simulink model "indi_controller_tuning"  (R2024b)
settings: Solver=FixedStepAuto  StartTime=0.0  StopTime=inf  FixedStep=0.001  RelTol=1e-3
undefined symbols (not defined in the file): dirty_derivative, drawaircraft, drawaircraft2, dspblkCoreblockFVToolHelper, force_moment, gcbh, INDI, MAV, position_rhombus, reference_model, sample_time, SIM
libraries: slpidlib x12
(part 2 of 2)

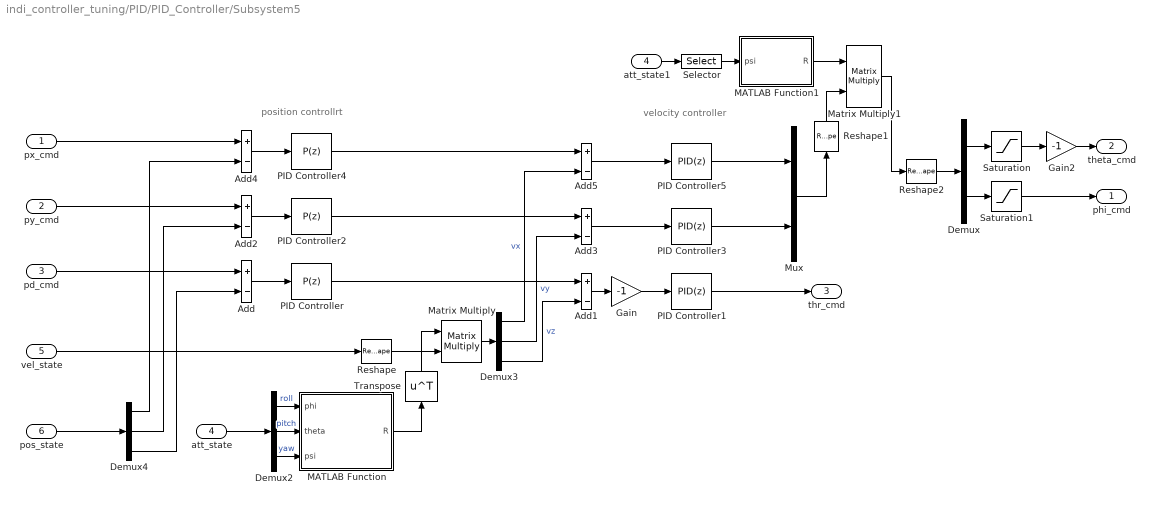
== system indi_controller_tuning/PID/PID_Controller/Subsystem5 ==
  note: velocity controller
  note: position controllrt
  px_cmd : Inport
  py_cmd : Inport  Port=2
  pd_cmd : Inport  Port=3
  att_state : Inport  Port=4
  vel_state : Inport  Port=5
  pos_state : Inport  Port=6
  Add{,1..5} (6 alike) : Sum  Inputs=+-
  Demux : Demux  Outputs=2
  Demux2 : Demux  Outputs=3
  Demux3 : Demux  Outputs=3
  Demux4 : Demux  Outputs=3
  Gain : Gain  Gain=-1
  Gain2 : Gain  Gain=-1
  MATLAB Function : MATLAB Function  TreatAsAtomicUnit=on
  MATLAB Function1 : MATLAB Function  TreatAsAtomicUnit=on
  Matrix Multiply : Product  Multiplication=Matrix(*)
  Matrix Multiply1 : Product  Multiplication=Matrix(*)
  Mux : Mux  Inputs=2
  PID Controller : slpidlib/PID Controller  Controller=P  Form=Parallel  TimeDomain=Discrete-time  UseExternalTs=off  SampleTime=sample_time  IntegratorMethod=Forward Euler  FilterMethod=Forward Euler  ControllerParametersSource=internal  P=1.55741678828513  I=1  UseKiTs=off  D=0  UseExternalDerivativeSource=off  N=100  UseFilter=on  TunerSelectOption=Transfer Function Based (PID Tuner App)  InitialConditionSource=internal  InitialConditionForIntegrator=0  InitialConditionForFilter=0  DifferentiatorICPrevScaledInput=0  ExternalReset=none  TrackingMode=off  Kt=1  LimitOutput=on  SatLimitsSource=internal  UpperSaturationLimit=2.5  LowerSaturationLimit=-2.5  LinearizeAsGain=on  AntiWindupMode=none  Kb=1  LimitIntegrator=off  UpperIntegratorSaturationLimit=inf  LowerIntegratorSaturationLimit=-inf  POutMin=[]  POutMax=[]  IOutMin=[]  IOutMax=[]  DOutMin=[]  DOutMax=[]  NOutMin=[]  NOutMax=[]  SumOutMin=[]  SumOutMax=[]  SaturationOutMin=[]  SaturationOutMax=[]  PParamMin=[]  PParamMax=[]  IParamMin=[]  IParamMax=[]  DParamMin=[]  DParamMax=[]  NParamMin=[]  NParamMax=[]  KbParamMin=[]  KbParamMax=[]  KtParamMin=[]  KtParamMax=[]  KbOutMin=[]  KbOutMax=[]  KtOutMin=[]  KtOutMax=[]  IntegratorOutMin=[]  IntegratorOutMax=[]  FilterOutMin=[]  FilterOutMax=[]  SumI1OutMin=[]  SumI1OutMax=[]  SumI2OutMin=[]  SumI2OutMax=[]  SumI3OutMin=[]  SumI3OutMax=[]  SumI4OutMin=[]  SumI4OutMax=[]  SumDOutMin=[]  SumDOutMax=[]  DifferentiatorOutMin=[]  DifferentiatorOutMax=[]  FilterDiffOutCoefMin=[]  FilterDiffOutCoefMax=[]  ReciprocalOutMin=[]  ReciprocalOutMax=[]  SumDenOutMin=[]  SumDenOutMax=[]  SumNumOutMin=[]  SumNumOutMax=[]  DivideOutMin=[]  DivideOutMax=[]  UdiffTsProdOutMin=[]  UdiffTsProdOutMax=[]  NTsProdOutMin=[]  NTsProdOutMax=[]  UintegralTsProdOutMin=[]  UintegralTsProdOutMax=[]  UngainTsProdOutMin=[]  UngainTsProdOutMax=[]  ClampingZeroOutDataTypeStr=Inherit: Inherit via back propagation  ClampingZeroOutMin=[]  ClampingZeroOutMax=[]  FilterDenConstantOutDataTypeStr=Inherit: Inherit via back propagation  FilterDenConstantOutMin=[]  FilterDenConstantOutMax=[]  PCopyOutDataTypeStr=Inherit: Inherit via back propagation  PCopyOutMin=[]  PCopyOutMax=[]  NCopyOutDataTypeStr=Inherit: Inherit via back propagation  NCopyOutMin=[]  NCopyOutMax=[]  IntegratorContinuousStateAttributes=''  IntegratorStateMustResolveToSignalObject=off  IntegratorRTWStateStorageClass=Auto  FilterContinuousStateAttributes=''  FilterStateMustResolveToSignalObject=off  FilterRTWStateStorageClass=Auto  ParallelPVariant=InternalParameters  IdealPVariant=Disabled  IVariant=Disabled  DVariant=Disabled  IntegratorVariant=Disabled  SatVariant=Enabled  AWVariant=Disabled  PCopyVariant=Disabled  TRVariant=Disabled  FdbkBlocksVariant=Forward  IdealPFdbkVariant=Disabled  SatFdbkVariant=Disabled  DerivativeFilterVariant=Disabled  NVariant=Disabled  NCopyVariant=Disabled_SignalSpec  FilterICVariant=Disabled  IntegratorICVariant=Disabled  ExternalResetVariant=Disabled  TRSumVariant=Passthrough  SumFdbkVariant=Disabled  SumVariant=Passthrough_P  TsampFilterVariant=InternalTs  TsampNgainVariant=Passthrough  TsampIntegralVariant=Disabled_SignalSpec  ExternalSaturationOutDataTypeStr=Inherit: Same as second input  DerivativeSourceVariant=Disabled  PreIntVariant=InternalPreInt
  PID Controller1 : slpidlib/PID Controller  Controller=PID  Form=Parallel  TimeDomain=Discrete-time  UseExternalTs=off  SampleTime=sample_time  IntegratorMethod=Forward Euler  FilterMethod=Forward Euler  ControllerParametersSource=internal  P=8.52067722160773  I=8.12576415570105  UseKiTs=off  D=0.164011038210978  UseExternalDerivativeSource=off  N=48.9353550982802  UseFilter=on  TunerSelectOption=Transfer Function Based (PID Tuner App)  InitialConditionSource=internal  InitialConditionForIntegrator=0  InitialConditionForFilter=0  DifferentiatorICPrevScaledInput=0  ExternalReset=none  TrackingMode=off  Kt=1  LimitOutput=on  SatLimitsSource=internal  UpperSaturationLimit=0.3*11  LowerSaturationLimit=-0.3*11  LinearizeAsGain=on  AntiWindupMode=clamping  Kb=1  LimitIntegrator=off  UpperIntegratorSaturationLimit=inf  LowerIntegratorSaturationLimit=-inf  POutMin=[]  POutMax=[]  IOutMin=[]  IOutMax=[]  DOutMin=[]  DOutMax=[]  NOutMin=[]  NOutMax=[]  SumOutMin=[]  SumOutMax=[]  SaturationOutMin=[]  SaturationOutMax=[]  PParamMin=[]  PParamMax=[]  IParamMin=[]  IParamMax=[]  DParamMin=[]  DParamMax=[]  NParamMin=[]  NParamMax=[]  KbParamMin=[]  KbParamMax=[]  KtParamMin=[]  KtParamMax=[]  KbOutMin=[]  KbOutMax=[]  KtOutMin=[]  KtOutMax=[]  IntegratorOutMin=[]  IntegratorOutMax=[]  FilterOutMin=[]  FilterOutMax=[]  SumI1OutMin=[]  SumI1OutMax=[]  SumI2OutMin=[]  SumI2OutMax=[]  SumI3OutMin=[]  SumI3OutMax=[]  SumI4OutMin=[]  SumI4OutMax=[]  SumDOutMin=[]  SumDOutMax=[]  DifferentiatorOutMin=[]  DifferentiatorOutMax=[]  FilterDiffOutCoefMin=[]  FilterDiffOutCoefMax=[]  ReciprocalOutMin=[]  ReciprocalOutMax=[]  SumDenOutMin=[]  SumDenOutMax=[]  SumNumOutMin=[]  SumNumOutMax=[]  DivideOutMin=[]  DivideOutMax=[]  UdiffTsProdOutMin=[]  UdiffTsProdOutMax=[]  NTsProdOutMin=[]  NTsProdOutMax=[]  UintegralTsProdOutMin=[]  UintegralTsProdOutMax=[]  UngainTsProdOutMin=[]  UngainTsProdOutMax=[]  ClampingZeroOutDataTypeStr=Inherit: Inherit via back propagation  ClampingZeroOutMin=[]  ClampingZeroOutMax=[]  FilterDenConstantOutDataTypeStr=Inherit: Inherit via back propagation  FilterDenConstantOutMin=[]  FilterDenConstantOutMax=[]  PCopyOutDataTypeStr=Inherit: Inherit via back propagation  PCopyOutMin=[]  PCopyOutMax=[]  NCopyOutDataTypeStr=Inherit: Inherit via back propagation  NCopyOutMin=[]  NCopyOutMax=[]  IntegratorContinuousStateAttributes=''  IntegratorStateMustResolveToSignalObject=off  IntegratorRTWStateStorageClass=Auto  FilterContinuousStateAttributes=''  FilterStateMustResolveToSignalObject=off  FilterRTWStateStorageClass=Auto  ParallelPVariant=InternalParameters  IdealPVariant=Disabled  IVariant=InternalParameters  DVariant=InternalParameters  IntegratorVariant=Discrete  SatVariant=Enabled  AWVariant=DiscClampingParallel  PCopyVariant=Disabled  TRVariant=Disabled  FdbkBlocksVariant=Forward  IdealPFdbkVariant=Disabled  SatFdbkVariant=Disabled  DerivativeFilterVariant=ForwardEulerFilter  NVariant=InternalParameters  NCopyVariant=Disabled  FilterICVariant=InternalICsFilter  IntegratorICVariant=InternalICs  ExternalResetVariant=Disabled  TRSumVariant=Passthrough  SumFdbkVariant=Disabled  SumVariant=Sum_PID  TsampFilterVariant=InternalTs  TsampNgainVariant=Passthrough  TsampIntegralVariant=Disabled_SignalSpec  ExternalSaturationOutDataTypeStr=Inherit: Same as second input  DerivativeSourceVariant=ErrorSignal  PreIntVariant=InternalPreInt
  PID Controller2 : slpidlib/PID Controller  Controller=P  Form=Parallel  TimeDomain=Discrete-time  UseExternalTs=off  SampleTime=sample_time  IntegratorMethod=Forward Euler  FilterMethod=Forward Euler  ControllerParametersSource=internal  P=0.183831516601899  I=1  UseKiTs=off  D=0  UseExternalDerivativeSource=off  N=100  UseFilter=on  TunerSelectOption=Transfer Function Based (PID Tuner App)  InitialConditionSource=internal  InitialConditionForIntegrator=0  InitialConditionForFilter=0  DifferentiatorICPrevScaledInput=0  ExternalReset=none  TrackingMode=off  Kt=1  LimitOutput=on  SatLimitsSource=internal  UpperSaturationLimit=5  LowerSaturationLimit=-5  LinearizeAsGain=on  AntiWindupMode=none  Kb=1  LimitIntegrator=off  UpperIntegratorSaturationLimit=inf  LowerIntegratorSaturationLimit=-inf  POutMin=[]  POutMax=[]  IOutMin=[]  IOutMax=[]  DOutMin=[]  DOutMax=[]  NOutMin=[]  NOutMax=[]  SumOutMin=[]  SumOutMax=[]  SaturationOutMin=[]  SaturationOutMax=[]  PParamMin=[]  PParamMax=[]  IParamMin=[]  IParamMax=[]  DParamMin=[]  DParamMax=[]  NParamMin=[]  NParamMax=[]  KbParamMin=[]  KbParamMax=[]  KtParamMin=[]  KtParamMax=[]  KbOutMin=[]  KbOutMax=[]  KtOutMin=[]  KtOutMax=[]  IntegratorOutMin=[]  IntegratorOutMax=[]  FilterOutMin=[]  FilterOutMax=[]  SumI1OutMin=[]  SumI1OutMax=[]  SumI2OutMin=[]  SumI2OutMax=[]  SumI3OutMin=[]  SumI3OutMax=[]  SumI4OutMin=[]  SumI4OutMax=[]  SumDOutMin=[]  SumDOutMax=[]  DifferentiatorOutMin=[]  DifferentiatorOutMax=[]  FilterDiffOutCoefMin=[]  FilterDiffOutCoefMax=[]  ReciprocalOutMin=[]  ReciprocalOutMax=[]  SumDenOutMin=[]  SumDenOutMax=[]  SumNumOutMin=[]  SumNumOutMax=[]  DivideOutMin=[]  DivideOutMax=[]  UdiffTsProdOutMin=[]  UdiffTsProdOutMax=[]  NTsProdOutMin=[]  NTsProdOutMax=[]  UintegralTsProdOutMin=[]  UintegralTsProdOutMax=[]  UngainTsProdOutMin=[]  UngainTsProdOutMax=[]  ClampingZeroOutDataTypeStr=Inherit: Inherit via back propagation  ClampingZeroOutMin=[]  ClampingZeroOutMax=[]  FilterDenConstantOutDataTypeStr=Inherit: Inherit via back propagation  FilterDenConstantOutMin=[]  FilterDenConstantOutMax=[]  PCopyOutDataTypeStr=Inherit: Inherit via back propagation  PCopyOutMin=[]  PCopyOutMax=[]  NCopyOutDataTypeStr=Inherit: Inherit via back propagation  NCopyOutMin=[]  NCopyOutMax=[]  IntegratorContinuousStateAttributes=''  IntegratorStateMustResolveToSignalObject=off  IntegratorRTWStateStorageClass=Auto  FilterContinuousStateAttributes=''  FilterStateMustResolveToSignalObject=off  FilterRTWStateStorageClass=Auto  ParallelPVariant=InternalParameters  IdealPVariant=Disabled  IVariant=Disabled  DVariant=Disabled  IntegratorVariant=Disabled  SatVariant=Enabled  AWVariant=Disabled  PCopyVariant=Disabled  TRVariant=Disabled  FdbkBlocksVariant=Forward  IdealPFdbkVariant=Disabled  SatFdbkVariant=Disabled  DerivativeFilterVariant=Disabled  NVariant=Disabled  NCopyVariant=Disabled_SignalSpec  FilterICVariant=Disabled  IntegratorICVariant=Disabled  ExternalResetVariant=Disabled  TRSumVariant=Passthrough  SumFdbkVariant=Disabled  SumVariant=Passthrough_P  TsampFilterVariant=InternalTs  TsampNgainVariant=Passthrough  TsampIntegralVariant=Disabled_SignalSpec  ExternalSaturationOutDataTypeStr=Inherit: Same as second input  DerivativeSourceVariant=Disabled  PreIntVariant=InternalPreInt
  PID Controller3 : slpidlib/PID Controller  Controller=PID  Form=Parallel  TimeDomain=Discrete-time  UseExternalTs=off  SampleTime=sample_time  IntegratorMethod=Forward Euler  FilterMethod=Forward Euler  ControllerParametersSource=internal  P=0.0381310436212984  I=0.0014813668367107  UseKiTs=off  D=-0.018399108574611  UseExternalDerivativeSource=off  N=1.45342970874378  UseFilter=on  TunerSelectOption=Transfer Function Based (PID Tuner App)  InitialConditionSource=internal  InitialConditionForIntegrator=0  InitialConditionForFilter=0  DifferentiatorICPrevScaledInput=0  ExternalReset=none  TrackingMode=off  Kt=1  LimitOutput=on  SatLimitsSource=internal  UpperSaturationLimit=deg2rad(8)  LowerSaturationLimit=-deg2rad(8)  LinearizeAsGain=on  AntiWindupMode=clamping  Kb=1  LimitIntegrator=off  UpperIntegratorSaturationLimit=inf  LowerIntegratorSaturationLimit=-inf  RndMeth=Ceiling  POutMin=[]  POutMax=[]  IOutMin=[]  IOutMax=[]  DOutMin=[]  DOutMax=[]  NOutMin=[]  NOutMax=[]  SumOutMin=[]  SumOutMax=[]  SaturationOutMin=[]  SaturationOutMax=[]  PParamMin=[]  PParamMax=[]  IParamMin=[]  IParamMax=[]  DParamMin=[]  DParamMax=[]  NParamMin=[]  NParamMax=[]  KbParamMin=[]  KbParamMax=[]  KtParamMin=[]  KtParamMax=[]  KbOutMin=[]  KbOutMax=[]  KtOutMin=[]  KtOutMax=[]  IntegratorOutMin=[]  IntegratorOutMax=[]  FilterOutMin=[]  FilterOutMax=[]  SumI1OutMin=[]  SumI1OutMax=[]  SumI2OutMin=[]  SumI2OutMax=[]  SumI3OutMin=[]  SumI3OutMax=[]  SumI4OutMin=[]  SumI4OutMax=[]  SumDOutMin=[]  SumDOutMax=[]  DifferentiatorOutMin=[]  DifferentiatorOutMax=[]  FilterDiffOutCoefMin=[]  FilterDiffOutCoefMax=[]  ReciprocalOutMin=[]  ReciprocalOutMax=[]  SumDenOutMin=[]  SumDenOutMax=[]  SumNumOutMin=[]  SumNumOutMax=[]  DivideOutMin=[]  DivideOutMax=[]  UdiffTsProdOutMin=[]  UdiffTsProdOutMax=[]  NTsProdOutMin=[]  NTsProdOutMax=[]  UintegralTsProdOutMin=[]  UintegralTsProdOutMax=[]  UngainTsProdOutMin=[]  UngainTsProdOutMax=[]  ClampingZeroOutDataTypeStr=Inherit: Inherit via back propagation  ClampingZeroOutMin=[]  ClampingZeroOutMax=[]  FilterDenConstantOutDataTypeStr=Inherit: Inherit via back propagation  FilterDenConstantOutMin=[]  FilterDenConstantOutMax=[]  PCopyOutDataTypeStr=Inherit: Inherit via back propagation  PCopyOutMin=[]  PCopyOutMax=[]  NCopyOutDataTypeStr=Inherit: Inherit via back propagation  NCopyOutMin=[]  NCopyOutMax=[]  IntegratorContinuousStateAttributes=''  IntegratorStateMustResolveToSignalObject=off  IntegratorRTWStateStorageClass=Auto  FilterContinuousStateAttributes=''  FilterStateMustResolveToSignalObject=off  FilterRTWStateStorageClass=Auto  ParallelPVariant=InternalParameters  IdealPVariant=Disabled  IVariant=InternalParameters  DVariant=InternalParameters  IntegratorVariant=Discrete  SatVariant=Enabled  AWVariant=DiscClampingParallel  PCopyVariant=Disabled  TRVariant=Disabled  FdbkBlocksVariant=Forward  IdealPFdbkVariant=Disabled  SatFdbkVariant=Disabled  DerivativeFilterVariant=ForwardEulerFilter  NVariant=InternalParameters  NCopyVariant=Disabled  FilterICVariant=InternalICsFilter  IntegratorICVariant=InternalICs  ExternalResetVariant=Disabled  TRSumVariant=Passthrough  SumFdbkVariant=Disabled  SumVariant=Sum_PID  TsampFilterVariant=InternalTs  TsampNgainVariant=Passthrough  TsampIntegralVariant=Disabled_SignalSpec  ExternalSaturationOutDataTypeStr=Inherit: Same as second input  DerivativeSourceVariant=ErrorSignal  PreIntVariant=InternalPreInt
  PID Controller4 : slpidlib/PID Controller  Controller=P  Form=Parallel  TimeDomain=Discrete-time  UseExternalTs=off  SampleTime=sample_time  IntegratorMethod=Forward Euler  FilterMethod=Forward Euler  ControllerParametersSource=internal  P=0.183831516601899  I=1  UseKiTs=off  D=0  UseExternalDerivativeSource=off  N=100  UseFilter=on  TunerSelectOption=Transfer Function Based (PID Tuner App)  InitialConditionSource=internal  InitialConditionForIntegrator=0  InitialConditionForFilter=0  DifferentiatorICPrevScaledInput=0  ExternalReset=none  TrackingMode=off  Kt=1  LimitOutput=on  SatLimitsSource=internal  UpperSaturationLimit=5  LowerSaturationLimit=-5  LinearizeAsGain=on  AntiWindupMode=none  Kb=1  LimitIntegrator=off  UpperIntegratorSaturationLimit=inf  LowerIntegratorSaturationLimit=-inf  POutMin=[]  POutMax=[]  IOutMin=[]  IOutMax=[]  DOutMin=[]  DOutMax=[]  NOutMin=[]  NOutMax=[]  SumOutMin=[]  SumOutMax=[]  SaturationOutMin=[]  SaturationOutMax=[]  PParamMin=[]  PParamMax=[]  IParamMin=[]  IParamMax=[]  DParamMin=[]  DParamMax=[]  NParamMin=[]  NParamMax=[]  KbParamMin=[]  KbParamMax=[]  KtParamMin=[]  KtParamMax=[]  KbOutMin=[]  KbOutMax=[]  KtOutMin=[]  KtOutMax=[]  IntegratorOutMin=[]  IntegratorOutMax=[]  FilterOutMin=[]  FilterOutMax=[]  SumI1OutMin=[]  SumI1OutMax=[]  SumI2OutMin=[]  SumI2OutMax=[]  SumI3OutMin=[]  SumI3OutMax=[]  SumI4OutMin=[]  SumI4OutMax=[]  SumDOutMin=[]  SumDOutMax=[]  DifferentiatorOutMin=[]  DifferentiatorOutMax=[]  FilterDiffOutCoefMin=[]  FilterDiffOutCoefMax=[]  ReciprocalOutMin=[]  ReciprocalOutMax=[]  SumDenOutMin=[]  SumDenOutMax=[]  SumNumOutMin=[]  SumNumOutMax=[]  DivideOutMin=[]  DivideOutMax=[]  UdiffTsProdOutMin=[]  UdiffTsProdOutMax=[]  NTsProdOutMin=[]  NTsProdOutMax=[]  UintegralTsProdOutMin=[]  UintegralTsProdOutMax=[]  UngainTsProdOutMin=[]  UngainTsProdOutMax=[]  ClampingZeroOutDataTypeStr=Inherit: Inherit via back propagation  ClampingZeroOutMin=[]  ClampingZeroOutMax=[]  FilterDenConstantOutDataTypeStr=Inherit: Inherit via back propagation  FilterDenConstantOutMin=[]  FilterDenConstantOutMax=[]  PCopyOutDataTypeStr=Inherit: Inherit via back propagation  PCopyOutMin=[]  PCopyOutMax=[]  NCopyOutDataTypeStr=Inherit: Inherit via back propagation  NCopyOutMin=[]  NCopyOutMax=[]  IntegratorContinuousStateAttributes=''  IntegratorStateMustResolveToSignalObject=off  IntegratorRTWStateStorageClass=Auto  FilterContinuousStateAttributes=''  FilterStateMustResolveToSignalObject=off  FilterRTWStateStorageClass=Auto  ParallelPVariant=InternalParameters  IdealPVariant=Disabled  IVariant=Disabled  DVariant=Disabled  IntegratorVariant=Disabled  SatVariant=Enabled  AWVariant=Disabled  PCopyVariant=Disabled  TRVariant=Disabled  FdbkBlocksVariant=Forward  IdealPFdbkVariant=Disabled  SatFdbkVariant=Disabled  DerivativeFilterVariant=Disabled  NVariant=Disabled  NCopyVariant=Disabled_SignalSpec  FilterICVariant=Disabled  IntegratorICVariant=Disabled  ExternalResetVariant=Disabled  TRSumVariant=Passthrough  SumFdbkVariant=Disabled  SumVariant=Passthrough_P  TsampFilterVariant=InternalTs  TsampNgainVariant=Passthrough  TsampIntegralVariant=Disabled_SignalSpec  ExternalSaturationOutDataTypeStr=Inherit: Same as second input  DerivativeSourceVariant=Disabled  PreIntVariant=InternalPreInt
  PID Controller5 : slpidlib/PID Controller  Controller=PID  Form=Parallel  TimeDomain=Discrete-time  UseExternalTs=off  SampleTime=sample_time  IntegratorMethod=Forward Euler  FilterMethod=Forward Euler  ControllerParametersSource=internal  P=0.0381310436212984  I=0.0014813668367107  UseKiTs=off  D=-0.018399108574611  UseExternalDerivativeSource=off  N=1.45342970874378  UseFilter=on  TunerSelectOption=Transfer Function Based (PID Tuner App)  InitialConditionSource=internal  InitialConditionForIntegrator=0  InitialConditionForFilter=0  DifferentiatorICPrevScaledInput=0  ExternalReset=none  TrackingMode=off  Kt=1  LimitOutput=on  SatLimitsSource=internal  UpperSaturationLimit=deg2rad(8)  LowerSaturationLimit=-deg2rad(8)  LinearizeAsGain=on  AntiWindupMode=clamping  Kb=1  LimitIntegrator=off  UpperIntegratorSaturationLimit=inf  LowerIntegratorSaturationLimit=-inf  RndMeth=Ceiling  POutMin=[]  POutMax=[]  IOutMin=[]  IOutMax=[]  DOutMin=[]  DOutMax=[]  NOutMin=[]  NOutMax=[]  SumOutMin=[]  SumOutMax=[]  SaturationOutMin=[]  SaturationOutMax=[]  PParamMin=[]  PParamMax=[]  IParamMin=[]  IParamMax=[]  DParamMin=[]  DParamMax=[]  NParamMin=[]  NParamMax=[]  KbParamMin=[]  KbParamMax=[]  KtParamMin=[]  KtParamMax=[]  KbOutMin=[]  KbOutMax=[]  KtOutMin=[]  KtOutMax=[]  IntegratorOutMin=[]  IntegratorOutMax=[]  FilterOutMin=[]  FilterOutMax=[]  SumI1OutMin=[]  SumI1OutMax=[]  SumI2OutMin=[]  SumI2OutMax=[]  SumI3OutMin=[]  SumI3OutMax=[]  SumI4OutMin=[]  SumI4OutMax=[]  SumDOutMin=[]  SumDOutMax=[]  DifferentiatorOutMin=[]  DifferentiatorOutMax=[]  FilterDiffOutCoefMin=[]  FilterDiffOutCoefMax=[]  ReciprocalOutMin=[]  ReciprocalOutMax=[]  SumDenOutMin=[]  SumDenOutMax=[]  SumNumOutMin=[]  SumNumOutMax=[]  DivideOutMin=[]  DivideOutMax=[]  UdiffTsProdOutMin=[]  UdiffTsProdOutMax=[]  NTsProdOutMin=[]  NTsProdOutMax=[]  UintegralTsProdOutMin=[]  UintegralTsProdOutMax=[]  UngainTsProdOutMin=[]  UngainTsProdOutMax=[]  ClampingZeroOutDataTypeStr=Inherit: Inherit via back propagation  ClampingZeroOutMin=[]  ClampingZeroOutMax=[]  FilterDenConstantOutDataTypeStr=Inherit: Inherit via back propagation  FilterDenConstantOutMin=[]  FilterDenConstantOutMax=[]  PCopyOutDataTypeStr=Inherit: Inherit via back propagation  PCopyOutMin=[]  PCopyOutMax=[]  NCopyOutDataTypeStr=Inherit: Inherit via back propagation  NCopyOutMin=[]  NCopyOutMax=[]  IntegratorContinuousStateAttributes=''  IntegratorStateMustResolveToSignalObject=off  IntegratorRTWStateStorageClass=Auto  FilterContinuousStateAttributes=''  FilterStateMustResolveToSignalObject=off  FilterRTWStateStorageClass=Auto  ParallelPVariant=InternalParameters  IdealPVariant=Disabled  IVariant=InternalParameters  DVariant=InternalParameters  IntegratorVariant=Discrete  SatVariant=Enabled  AWVariant=DiscClampingParallel  PCopyVariant=Disabled  TRVariant=Disabled  FdbkBlocksVariant=Forward  IdealPFdbkVariant=Disabled  SatFdbkVariant=Disabled  DerivativeFilterVariant=ForwardEulerFilter  NVariant=InternalParameters  NCopyVariant=Disabled  FilterICVariant=InternalICsFilter  IntegratorICVariant=InternalICs  ExternalResetVariant=Disabled  TRSumVariant=Passthrough  SumFdbkVariant=Disabled  SumVariant=Sum_PID  TsampFilterVariant=InternalTs  TsampNgainVariant=Passthrough  TsampIntegralVariant=Disabled_SignalSpec  ExternalSaturationOutDataTypeStr=Inherit: Same as second input  DerivativeSourceVariant=ErrorSignal  PreIntVariant=InternalPreInt
  Reshape : Reshape  OutputDimensionality=Column vector (2-D)
  Reshape1 : Reshape  OutputDimensionality=Column vector (2-D)
  Reshape2 : Reshape  OutputDimensionality=Row vector (2-D)
  Saturation : Saturate  UpperLimit=deg2rad(6)  LowerLimit=-deg2rad(6)
  Saturation1 : Saturate  UpperLimit=deg2rad(6)  LowerLimit=-deg2rad(6)
  Selector : Selector  InputPortWidth=3  IndexOptions=Index vector (dialog)  Indices=[3]  OutputSizes=1
  Transpose : Math  Operator=transpose
  att_state1 : InportShadow  Port=4
  phi_cmd : Outport
  theta_cmd : Outport  Port=2
  thr_cmd : Outport  Port=3
  wires:
  Reshape/1 -> Matrix Multiply/2
  Demux3/3 -> Add1/2  "vz"
  Matrix Multiply/1 -> Demux3/1
  MATLAB Function/1(R) -> Transpose/1
  Add1/1 -> Gain/1
  Transpose/1 -> Matrix Multiply/1
  Demux2/1 -> MATLAB Function/1(phi)  "roll"
  Add/1 -> PID Controller/1
  Demux4/3 -> Add/2
  Demux2/3 -> MATLAB Function/3(psi)  "yaw"
  Demux2/2 -> MATLAB Function/2(theta)  "pitch"
  Gain/1 -> PID Controller1/1
  vel_state/1 -> Reshape/1
  pos_state/1 -> Demux4/1
  PID Controller1/1 -> thr_cmd/1
  att_state/1 -> Demux2/1
  pd_cmd/1 -> Add/1
  PID Controller/1 -> Add1/1
  Demux4/2 -> Add2/2
  py_cmd/1 -> Add2/1
  Demux3/2 -> Add3/2  "vy"
  Add3/1 -> PID Controller3/1
  Add2/1 -> PID Controller2/1
  Demux4/1 -> Add4/2
  px_cmd/1 -> Add4/1
  Add4/1 -> PID Controller4/1
  Add5/1 -> PID Controller5/1
  Demux3/1 -> Add5/2  "vx"
  Saturation1/1 -> phi_cmd/1
  Demux/1 -> Saturation/1
  Demux/2 -> Saturation1/1
  Reshape2/1 -> Demux/1
  Matrix Multiply1/1 -> Reshape2/1
  MATLAB Function1/1(R) -> Matrix Multiply1/1
  PID Controller3/1 -> Mux/2
  Saturation/1 -> Gain2/1
  att_state1/1 -> Selector/1
  Selector/1 -> MATLAB Function1/1(psi)
  PID Controller5/1 -> Mux/1
  Gain2/1 -> theta_cmd/1
  Mux/1 -> Reshape1/1
  Reshape1/1 -> Matrix Multiply1/2
  PID Controller4/1 -> Add5/1
  PID Controller2/1 -> Add3/1

== system indi_controller_tuning/PID/PID_Controller/control_allocation ==
  tau_roll : Inport
  tau_pitch : Inport  Port=2
  tau_yaw : Inport  Port=3
  thr_cmd : Inport  Port=4
  MATLAB Function : MATLAB Function  TreatAsAtomicUnit=on
  Reshape : Reshape  OutputDimensionality=Column vector (2-D)
  Selector : Selector  InputPortWidth=5  IndexOptions=Index vector (dialog)  Indices=[5]  OutputSizes=1
  Subsystem : Subsystem
  Unit Delay : UnitDelay  InitialCondition=0.7245  SampleTime=-1  HasFrameUpgradeWarning=on
  deltas : Outport
  wires:
  Reshape/1 -> MATLAB Function/1(fm)
  MATLAB Function/1(deltas) -> Selector/1, deltas/1
  tau_roll/1 -> Subsystem/1(taux)
  tau_pitch/1 -> Subsystem/2(tauy)
  thr_cmd/1 -> Subsystem/4(thr)
  Subsystem/1(cmd) -> Reshape/1
  tau_yaw/1 -> Subsystem/3(tauz)
  Unit Delay/1 -> MATLAB Function/2(prev_delt)
  Selector/1 -> Unit Delay/1

== system indi_controller_tuning/INDI/INDI_controller/trim_values/Subsystem1 ==
  Constant : Constant  Value=0.0
  Constant1 : Constant  Value=0.0
  Constant2 : Constant  Value=0.000998527156824563
  Constant3 : Constant  Value=8.4550 + 0.11
  Gain : Gain  Gain=-1
  Mux : Mux
  cmd : Outport
  wires:
  Mux/1 -> cmd/1
  Constant/1 -> Mux/1
  Gain/1 -> Mux/4
  Constant2/1 -> Mux/3
  Constant3/1 -> Gain/1
  Constant1/1 -> Mux/2

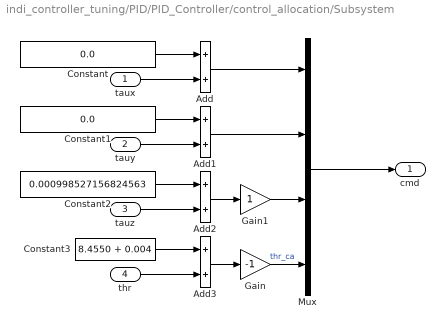
== system indi_controller_tuning/PID/PID_Controller/control_allocation/Subsystem ==
  taux : Inport
  tauy : Inport  Port=2
  tauz : Inport  Port=3
  thr : Inport  Port=4
  Add{,1..3} (4 alike) : Sum
  Constant : Constant  Value=0.0
  Constant1 : Constant  Value=0.0
  Constant2 : Constant  Value=0.000998527156824563
  Constant3 : Constant  Value=8.4550 + 0.004
  Gain : Gain  Gain=-1
  Gain1 : Gain
  Mux : Mux
  cmd : Outport
  wires:
  taux/1 -> Add/2
  Add2/1 -> Gain1/1
  Constant/1 -> Add/1
  Mux/1 -> cmd/1
  Add1/1 -> Mux/2
  Add/1 -> Mux/1
  Constant1/1 -> Add1/1
  tauy/1 -> Add1/2
  tauz/1 -> Add2/2
  Constant2/1 -> Add2/1
  Add3/1 -> Gain/1
  thr/1 -> Add3/2
  Constant3/1 -> Add3/1
  Gain/1 -> Mux/4  "thr_ca"
  Gain1/1 -> Mux/3

== matlab function indi_controller_tuning/PID/PID_Controller/Subsystem5/MATLAB Function1 ==
  data: psi input; R output
function R = R_psi(psi)
    R = [cos(psi), sin(psi);
        -sin(psi), cos(psi)];
end

== matlab function indi_controller_tuning/PID/PID_Controller/control_allocation/MATLAB Function ==
  data: fm input; deltas output; prev_delt input; MAV parameter
function deltas   = control_allocation(fm, prev_delt, MAV)
    % desired_forces_moments = [Mx; My; Mz; Fz]
    
    volt_prev = MAV.prop_data.volt_max * prev_delt;
    [T1, tau1] = prop_second_order(0, volt_prev, MAV);
    v_flap = sqrt(T1 / (2 * MAV.rho * MAV.prop_data.prop_area));
    
    q = 0.5 * MAV.rho * (v_flap^2); 
    C_lift = q * MAV.flap.s * MAV.flap.cla;
    
    K_T = T1 / prev_delt;
    K_Q = tau1 / prev_delt;

    % Mapping: [d1, d2, d3, d4, dt] -> [Mx, My, Mz, Fz]
    xt = MAV.flap.xt; yt = MAV.flap.yt; zt = MAV.flap.zt;
    
    B = [ ...
        (-zt*C_lift),  0,            (-zt*C_lift), 0,            0;
        0,             (-zt*C_lift), 0,            (-zt*C_lift), 0;
        (xt*C_lift),   (-yt*C_lift), (-xt*C_lift), (yt*C_lift),  K_Q;
        0,             0,            0,            0,            -K_T;
    ];
    
    % Pseudo Inverse
    P = pinv(B);
    
    % Raw Actuator Commands
    deltas = P * fm;
end

== matlab function indi_controller_tuning/PID/PID_Controller/Subsystem5/MATLAB Function ==
  data: phi input; R output; theta input; psi input
function R = rotate_inter2body(phi, theta, psi)
    R_psi = [cos(psi), sin(psi), 0;
            -sin(psi), cos(psi), 0
            0, 0, 1];
    R_theta = [cos(theta), 0, -sin(theta);
                0 , 1, 0;
                sin(theta), 0, cos(theta)];
    R_phi = [1, 0, 0;
             0, cos(phi), sin(phi);
             0, -sin(phi), cos(phi)];
    R = R_phi * R_theta * R_psi;
end

== matlab function indi_controller_tuning/INDI/INDI_controller/control_allocation/MATLAB Function ==
  data: fm input; deltas output; prev_delt input; MAV parameter
function deltas = control_allocation_indi(fm, prev_delt, MAV)
    % desired_forces_moments = [Mx; My; Mz; Fz] (Incremental)
    
    MIN_THROTTLE = 0.0;
    MAX_FLAP_RAD = 2 * pi / 180; 
    
    throttle_safe = max(prev_delt, 0.05);

    volt_prev = MAV.prop_data.volt_max * throttle_safe;
    [T1, tau1] = prop_second_order(0, volt_prev, MAV);
    if T1 < 0, T1 = 0; end
    
    v_flap = sqrt(T1 / (2 * MAV.rho * MAV.prop_data.prop_area));
    q = 0.5 * MAV.rho * (v_flap^2); 
    C_lift = q * MAV.flap.s * MAV.flap.cla;
    
    K_T = T1 / throttle_safe;
    K_Q = tau1 / throttle_safe;

    xt = MAV.flap.xt; yt = MAV.flap.yt; zt = MAV.flap.zt; 
   
    B = [ ...
        (-zt*C_lift),  0,            (-zt*C_lift), 0,            0;
        0,             (-zt*C_lift), 0,            (-zt*C_lift), 0;
        (xt*C_lift),   (-yt*C_lift), (-xt*C_lift), (yt*C_lift),  K_Q;
        0,             0,            0,            0,            -K_T;
    ];
    
    P = pinv(B);
    
    u_cmd = P * fm;

    flaps = max(min(u_cmd(1:4), MAX_FLAP_RAD), -MAX_FLAP_RAD);
    throttle_delta = u_cmd(5);
    
    deltas = [flaps; throttle_delta];
end

== matlab function indi_controller_tuning/INDI/INDI_controller/trim_values/MATLAB Function ==
  data: fm input; deltas output; prev_delt input; MAV parameter
function deltas   = control_allocation_indi(fm, prev_delt, MAV)
    % desired_forces_moments = [Mx; My; Mz; Fz]
    
    MIN_THROTTLE = 0.0;
    MAX_FLAP_RAD = 25 * pi / 180;
    
    volt_prev = MAV.prop_data.volt_max * prev_delt;
    [T1, tau1] = prop_second_order(0, volt_prev, MAV);
    if T1 < 0, T1 = 0; end
    v_flap = sqrt(T1 / (2 * MAV.rho * MAV.prop_data.prop_area));
    
    q = 0.5 * MAV.rho * (v_flap^2); 
    C_lift = q * MAV.flap.s * MAV.flap.cla;
    
    K_T = T1 / prev_delt;
    K_Q = tau1 / prev_delt;
    % Mapping: [d1, d2, d3, d4, dt] -> [Mx, My, Mz, Fz]
    xt = MAV.flap.xt; yt = MAV.flap.yt; zt = MAV.flap.zt; 
    % change in force (consistent with the change in the moment)
    del_f = fm(4,1) - T1;
   
    B = [ ...
        (-zt*C_lift),  0,            (-zt*C_lift), 0,            0;
        0,             (-zt*C_lift), 0,            (-zt*C_lift), 0;
        (xt*C_lift),   (-yt*C_lift), (-xt*C_lift), (yt*C_lift),  K_Q;
        0,             0,            0,            0,            -K_T;
    ];
    
    % Pseudo Inverse
    P = pinv(B);
    
    % Raw Actuator Commands
    % fm(4,1) = del_f; 
    
    u_cmd = P * fm;
    flaps = max(min(u_cmd(1:4), MAX_FLAP_RAD), -MAX_FLAP_RAD);
    throttle = u_cmd(5);
    % throttle = max(0, min(del_throttle + prev_delt,1));

    deltas = [flaps; throttle];
end
